simulink model "PED"  (R2020a)
settings: Solver=VariableStepAuto  StartTime=0.0  StopTime=10.0  RelTol=1e-3
settings Model: Creator=Marcus  LastModifiedBy=Marcus

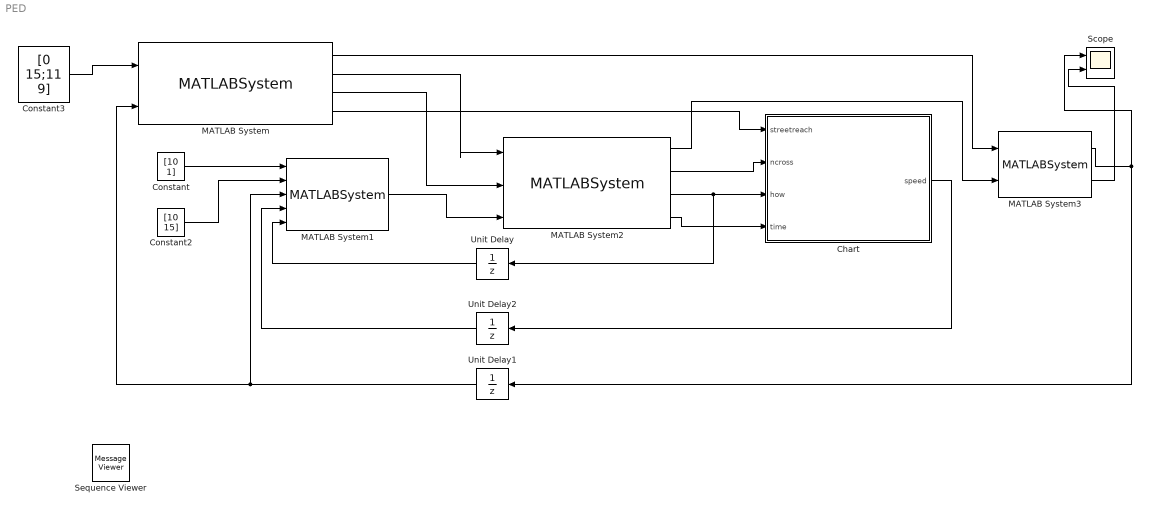
== system PED ==
  Chart : Stateflow chart  TreatAsAtomicUnit=on
  Constant : Constant  Value=[10 1]
  Constant2 : Constant  Value=[10 15]
  Constant3 : Constant  Value=[0 15;11 9]
  MATLAB System : MATLABSystem  System=environmentAwareness  SimulateUsing=Interpreted execution
      mask Type: environmentAwareness
      mask Display:
      | disp('environmentAwareness');
      | port_label('input',1,'carpos');
      | port_label('input',2,'pos');
      | port_label('output',1,'Carpos');
      | port_label('output',2,'closestcr');
      | port_label('output',3,'timegap');
      | port_label('output',4,'Streetreach');
  MATLAB System1 : MATLABSystem  System=trajPlanner  SimulateUsing=Interpreted execution
      mask Type: trajPlanner
      mask Display:
      | disp('trajPlanner');
      | port_label('input',1,'ipos');
      | port_label('input',2,'dpos');
      | port_label('input',3,'pos');
      | port_label('input',4,'speed');
      | port_label('input',5,'mustinclude');
      | port_label('output',1,'traj');
  MATLAB System2 : MATLABSystem  System=crossingbehavior  SimulateUsing=Interpreted execution
      mask Type: crossingbehavior
      mask Display:
      | disp('crossingbehavior');
      | port_label('input',1,'clocations');
      | port_label('input',2,'timegap');
      | port_label('input',3,'traj');
      | port_label('output',1,'npos');
      | port_label('output',2,'crossing');
      | port_label('output',3,'how');
      | port_label('output',4,'time');
  MATLAB System3 : MATLABSystem  System=forward  SimulateUsing=Interpreted execution
      mask Type: forward
      mask Display:
      | disp('forward');
      | port_label('input',1,'car');
      | port_label('input',2,'npos');
      | port_label('output',1,'pos');
      | port_label('output',2,'Car');
  Scope : Scope  NumInputPorts=2
  Sequence Viewer : MessageViewer  History=1000  SavedRootId=#
  Unit Delay : UnitDelay  SampleTime=-1  HasFrameUpgradeWarning=on
  Unit Delay1 : UnitDelay  SampleTime=-1  HasFrameUpgradeWarning=on
  Unit Delay2 : UnitDelay  SampleTime=-1  HasFrameUpgradeWarning=on
  wires:
  MATLAB System2/2 -> Chart/2(ncross)
  MATLAB System2/1 -> MATLAB System3/2
  MATLAB System3/1 -> Unit Delay1/1, Scope/1
  MATLAB System1/1 -> MATLAB System2/3
  MATLAB System/2 -> MATLAB System2/1
  MATLAB System/3 -> MATLAB System2/2
  Constant/1 -> MATLAB System1/1
  Unit Delay1/1 -> MATLAB System1/3, MATLAB System/2
  Chart/1(speed) -> Unit Delay2/1
  Unit Delay2/1 -> MATLAB System1/4
  Unit Delay/1 -> MATLAB System1/5
  Constant2/1 -> MATLAB System1/2
  Constant3/1 -> MATLAB System/1
  MATLAB System/1 -> MATLAB System3/1
  MATLAB System/4 -> Chart/1(streetreach)
  MATLAB System2/3 -> Unit Delay/1, Chart/3(how)
  MATLAB System2/4 -> Chart/4(time)
  MATLAB System3/2 -> Scope/2

== stateflow chart PED/Chart ==
  state Walk
    entry:
    fcross=false;
    during:
    speed=5
  state NeedToCross
    state WalkTowards
      speed=4;
    state Random
      state Stop
        entry:
        speed=0;
      state Go
        entry:
        speed=5;
      state Fast
        entry:
        speed=8;
      (default) -> NeedToCross.Random.Stop
      NeedToCross.Random.Stop -> NeedToCross.Random.Go : [time>=4]
      NeedToCross.Random.Go -> NeedToCross.Random.Fast : [time<=4]
      NeedToCross.Random.Fast -> NeedToCross.Random.Go
    state Zebra
      state Stop
        entry:
        speed=0;
      state Go
        entry:
        speed=5;
      (default) -> NeedToCross.Zebra.Stop
      NeedToCross.Zebra.Stop -> NeedToCross.Zebra.Go
    state Lights
      state Stop
        entry:
        speed=0;
      state Fast
        entry:
        speed=8;
      state Go
        entry:
        speed=5;
      (default) -> NeedToCross.Lights.Stop
      NeedToCross.Lights.Stop -> NeedToCross.Lights.Go
      NeedToCross.Lights.Go -> NeedToCross.Lights.Fast
      NeedToCross.Lights.Fast -> NeedToCross.Lights.Go
    state Finish
      during:
      fcross=true;
    (default) -> WalkTowards
    WalkTowards -> Random [order 1] : [streetreach==true & how==1]
    WalkTowards -> Lights [order 3] : [streetreach==true & how==3]
    WalkTowards -> Zebra [order 2] : [streetreach==true & how==2]
    Random -> Finish : [streetreach==false]
    Zebra -> Finish : [streetreach==false]
    Lights -> Finish : [streetreach==false]
  (default) -> Walk
  Walk -> NeedToCross : [ncross==true]
  NeedToCross -> Walk : [fcross==true]
  data: streetreach input; ncross input; how input; speed output; fcross local; time input
